simulink model "block_diagram"  (R2025b)
settings: Solver=VariableStepAuto  StartTime=0.0  StopTime=10.0  RelTol=1e-3
undefined symbols (not defined in the file): G1_den, G1_num, G2_den, G2_num, H_den, H_num, T_den, T_num
settings Model: Creator=nuris  LastModifiedBy=nuris

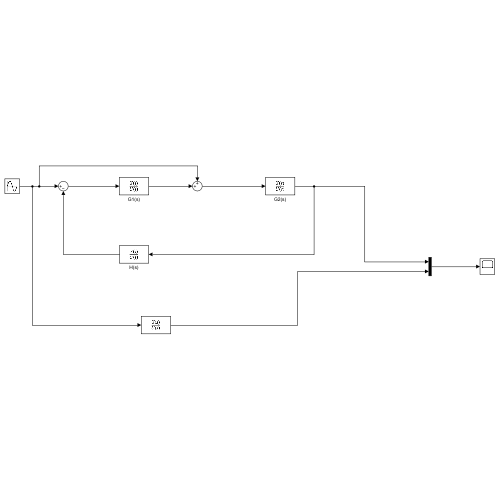
[thumbnail: Simulink's stored preview of the top-level diagram]
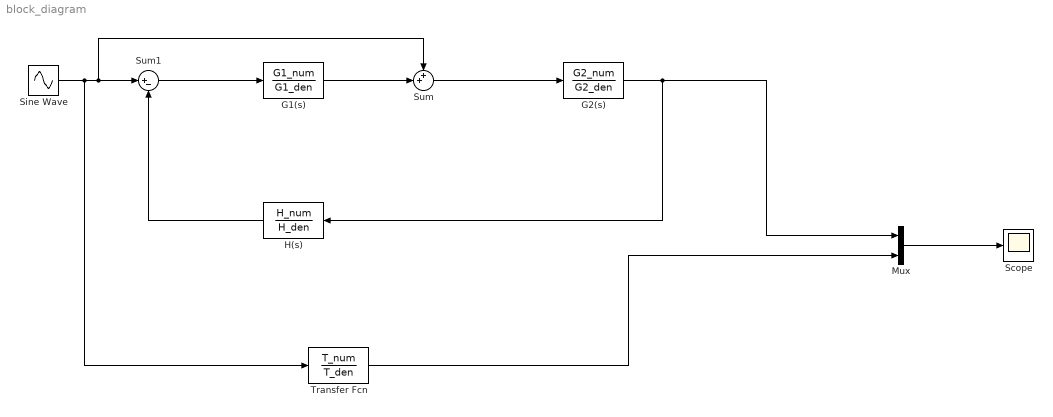
== system block_diagram ==
  G1(s) : TransferFcn  Numerator=G1_num  Denominator=G1_den
  G2(s) : TransferFcn  Numerator=G2_num  Denominator=G2_den
  H(s) : TransferFcn  Numerator=H_num  Denominator=H_den
  Mux : Mux  Inputs=2
  Scope : Scope
      settings: ActiveDisplayYMinimum=-0.2487319779509222  ActiveDisplayYMaximum=0.24367011526052287
  Sine Wave : Sin  SampleTime=0
  Sum : Sum  Inputs=++|
  Sum1 : Sum  Inputs=|+-
  Transfer Fcn : TransferFcn  Numerator=T_num  Denominator=T_den
  wires:
  G1(s)/1 -> Sum/2
  Sum1/1 -> G1(s)/1
  Sum/1 -> G2(s)/1
  H(s)/1 -> Sum1/2
  Sine Wave/1 -> Transfer Fcn/1, Sum/1, Sum1/1
  Transfer Fcn/1 -> Mux/2
  Mux/1 -> Scope/1
  G2(s)/1 -> H(s)/1, Mux/1
